simulink model "Controller"  (R2022b)
settings: Solver=FixedStepDiscrete  StartTime=0.0  StopTime=10.0  FixedStep=CONTROL_CONST.dt  MaxStep=CONTROL_PARAM.dt  RelTol=1e-3
values from neighbouring files (symbols this model uses):
  CONTROL_EXPORT = Simulink.Parameter(CONTROL_EXPORT_VALUE)    [control_model_init.m]
  CONTROL_PARAM = Simulink.Parameter(CONTROL_PARAM_VALUE)    [control_model_init.m]
undefined symbols (not defined in the file or in its folder): actuator_cmd, CONTROL_CONST, DiscIntNeverNeededParam, timestamp
libraries: simulink x3, FMT_Model_Lib x2, simulink_extras x2, drivingvehiclecontroller x2
settings Model: Creator=19114  LastModifiedBy=19114
settings OptimizationCC: DefaultParameterBehavior=Inlined  DefaultUnderspecifiedDataType=single  EnhancedBackFolding=on  PassReuseOutputArgsAs=Individual arguments  ZeroExternalMemoryAtStartup=off  ZeroInternalMemoryAtStartup=off  OptimizeBlockOrder=speed  DifferentSizesBufferReuse=on  OptimizationCustomize=off  EfficientTunableParamExpr=on
settings DebuggingCC: ParameterTunabilityLossMsg=error  UnconnectedInputMsg=warning  UnconnectedOutputMsg=warning  UnconnectedLineMsg=warning
settings HardwareCC: ProdBitPerPointer=32  ProdBitPerSizeT=32  ProdBitPerPtrDiffT=32  ProdLargestAtomicInteger=Long  ProdLargestAtomicFloat=Double  ProdWordSize=32  ProdHWDeviceType=ARM Compatible->ARM Cortex-M
settings ModelReferenceCC: EnableRefExpFcnMdlSchedulingChecks=on
settings SFSimCC: MATLABDynamicMemAlloc=off
settings RTWCC: Description=Embedded Coder  SystemTargetFile=ert.tlc  TemplateMakefile=ert_default_tmf  DLArmComputeVersion=19.05
settings CodeAppCC: ForceParamTrailComments=on  IgnoreCustomStorageClasses=off  OperatorAnnotations=on  SimulinkDataObjDesc=on  SFDataObjDesc=on  InsertBlockDesc=on
settings ERTTargetCC: TargetLangStandard=C99 (ISO)  GenerateSampleERTMain=on  SupportVariableSizeSignals=on  InlinedParameterPlacement=NonHierarchical  ERTCustomFileTemplate=example_file_process.tlc

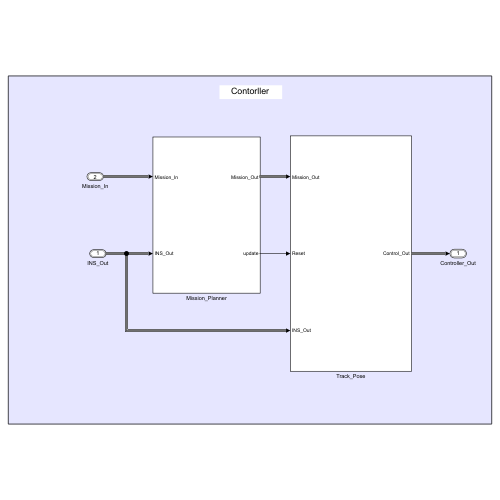
[thumbnail: Simulink's stored preview of the top-level diagram]
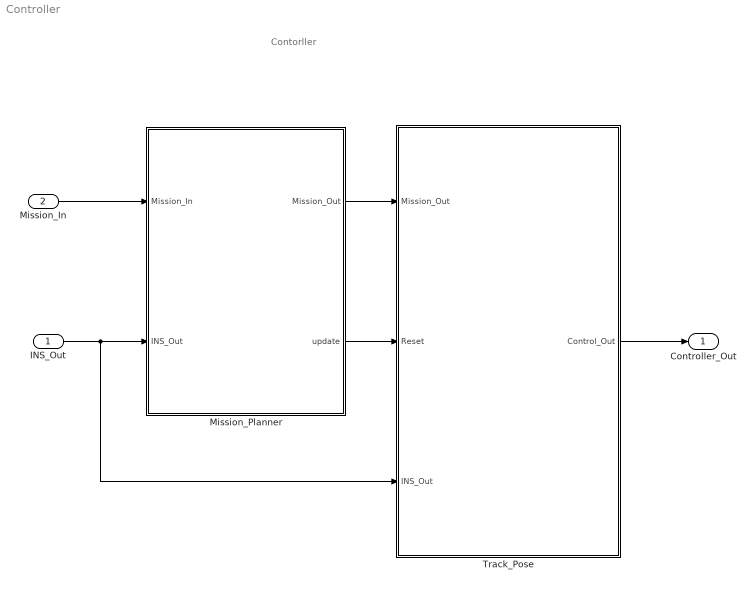
== system Controller ==
  note: Contorller
  INS_Out : Inport  OutDataTypeStr=Bus: INS_Out_Bus
  Mission_In : Inport  Port=2  OutDataTypeStr=Bus: Mission_Bus
  Mission_Planner : Subsystem
  Track_Pose : Subsystem
  Controller_Out : Outport  OutDataTypeStr=Bus: Control_Out_Bus
  wires:
  Track_Pose/1(Control_Out) -> Controller_Out/1
  Mission_Planner/1(Mission_Out) -> Track_Pose/1(Mission_Out)
  INS_Out/1 -> Mission_Planner/2(INS_Out), Track_Pose/3(INS_Out)
  Mission_In/1 -> Mission_Planner/1(Mission_In)
  Mission_Planner/2(update) -> Track_Pose/2(Reset)

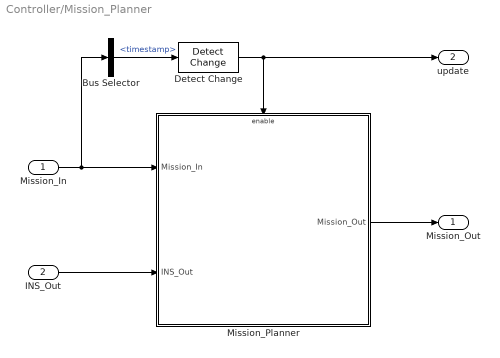
== system Controller/Mission_Planner ==
  Mission_In : Inport
  INS_Out : Inport  Port=2
  Bus Selector : BusSelector  OutputSignals=timestamp
  Detect Change : simulink/Logic and Bit Operations/Detect Change  vinit=0  OutDataTypeStr=boolean
  Mission_Planner : Subsystem
  Mission_Out : Outport
  update : Outport  Port=2
  wires:
  INS_Out/1 -> Mission_Planner/2(INS_Out)
  Mission_Planner/1(Mission_Out) -> Mission_Out/1
  Bus Selector/1 -> Detect Change/1  "<timestamp>"
  Mission_In/1 -> Bus Selector/1, Mission_Planner/1(Mission_In)
  Detect Change/1 -> Mission_Planner/Enable, update/1

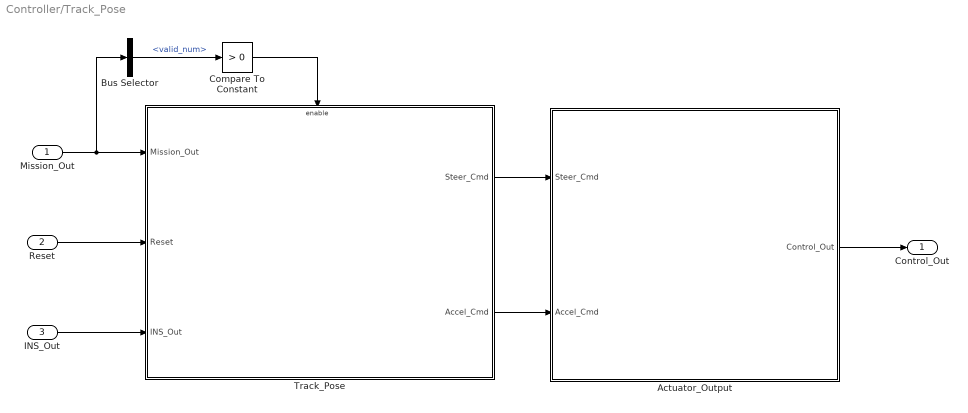
== system Controller/Track_Pose ==
  Mission_Out : Inport
  Reset : Inport  Port=2
  INS_Out : Inport  Port=3
  Actuator_Output : Subsystem
  Bus Selector : BusSelector  OutputSignals=valid_num
  Compare To Constant : simulink/Logic and Bit Operations/Compare To Constant  relop=>  const=0  OutDataTypeStr=boolean
  Track_Pose : Subsystem
  Control_Out : Outport
  wires:
  Reset/1 -> Track_Pose/2(Reset)
  Mission_Out/1 -> Bus Selector/1, Track_Pose/1(Mission_Out)
  INS_Out/1 -> Track_Pose/3(INS_Out)
  Bus Selector/1 -> Compare To Constant/1  "<valid_num>"
  Compare To Constant/1 -> Track_Pose/Enable
  Actuator_Output/1(Control_Out) -> Control_Out/1
  Track_Pose/1(Steer_Cmd) -> Actuator_Output/1(Steer_Cmd)
  Track_Pose/2(Accel_Cmd) -> Actuator_Output/2(Accel_Cmd)

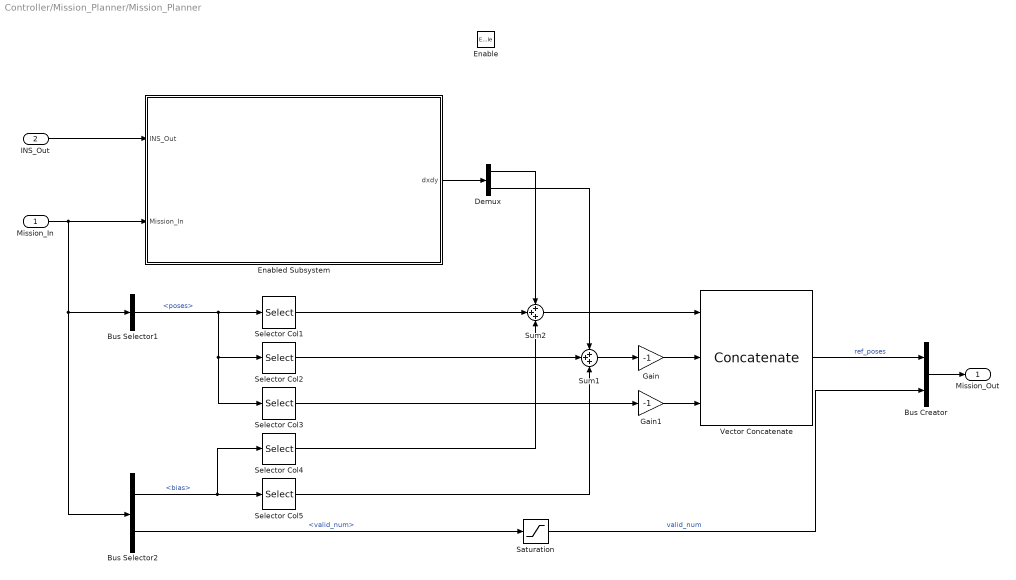
== system Controller/Mission_Planner/Mission_Planner ==
  Mission_In : Inport
  INS_Out : Inport  Port=2
  Enable : EnablePort
  Bus Creator : BusCreator  Inputs=2
  Bus Selector1 : BusSelector  OutputSignals=poses
  Bus Selector2 : BusSelector  OutputSignals=bias,valid_num
  Demux : Demux  Outputs=2
  Enabled Subsystem : Subsystem  TreatAsAtomicUnit=on
  Gain : Gain  Gain=-1
  Gain1 : Gain  Gain=-1
  Saturation : Saturate  UpperLimit=50  LowerLimit=0
  Selector Col1 : Selector  NumberOfDimensions=2  InputPortWidth=3  IndexOptions=Select all,Index vector (dialog)  Indices=[1 3],1  OutputSizes=1,1
  Selector Col2 : Selector  NumberOfDimensions=2  InputPortWidth=3  IndexOptions=Select all,Index vector (dialog)  Indices=[1 3],2  OutputSizes=1,1
  Selector Col3 : Selector  NumberOfDimensions=2  InputPortWidth=3  IndexOptions=Select all,Index vector (dialog)  Indices=[1 3],3  OutputSizes=1,1
  Selector Col4 : Selector  InputPortWidth=2  IndexOptions=Index vector (dialog)  Indices=[1]  OutputSizes=1
  Selector Col5 : Selector  InputPortWidth=2  IndexOptions=Index vector (dialog)  Indices=[1]  OutputSizes=1
  Sum1 : Sum  Inputs=+++
  Sum2 : Sum  Inputs=+++
  Vector Concatenate : Concatenate  NumInputs=3  Mode=Multidimensional array  ConcatenateDimension=2
  Mission_Out : Outport
  wires:
  Demux/1 -> Sum2/1
  Bus Selector1/1 -> Selector Col3/1, Selector Col2/1, Selector Col1/1  "<poses>"
  Demux/2 -> Sum1/1
  Selector Col3/1 -> Gain1/1
  Selector Col5/1 -> Sum1/3
  Bus Selector2/1 -> Selector Col4/1, Selector Col5/1  "<bias>"
  Mission_In/1 -> Bus Selector2/1, Bus Selector1/1, Enabled Subsystem/2(Mission_In)
  Saturation/1 -> Bus Creator/2  "valid_num"
  Vector Concatenate/1 -> Bus Creator/1  "ref_poses"
  Selector Col1/1 -> Sum2/2
  Enabled Subsystem/1(dxdy) -> Demux/1
  Selector Col2/1 -> Sum1/2
  Bus Selector2/2 -> Saturation/1  "<valid_num>"
  Selector Col4/1 -> Sum2/3
  Gain/1 -> Vector Concatenate/2
  Gain1/1 -> Vector Concatenate/3
  INS_Out/1 -> Enabled Subsystem/1(INS_Out)
  Sum1/1 -> Gain/1
  Sum2/1 -> Vector Concatenate/1
  Bus Creator/1 -> Mission_Out/1

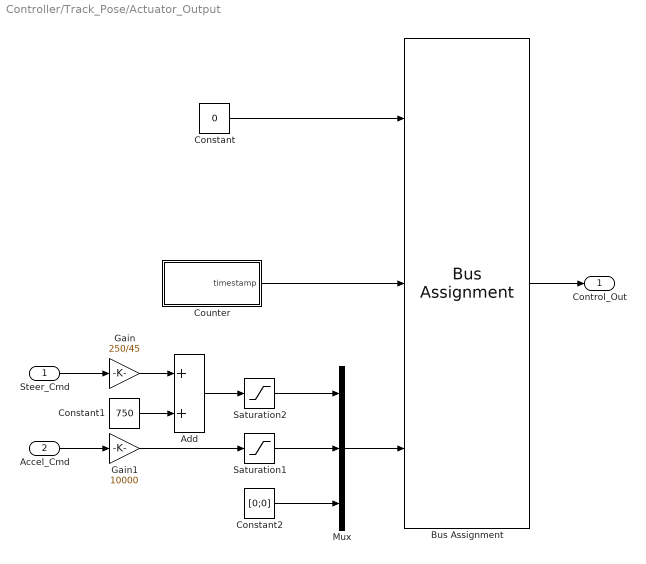
== system Controller/Track_Pose/Actuator_Output ==
  Steer_Cmd : Inport
  Accel_Cmd : Inport  Port=2
  Add : Sum
  Bus Assignment : BusAssignment  AssignedSignals=timestamp,actuator_cmd
  Constant : Constant  Value=0  OutDataTypeStr=Bus: Control_Out_Bus
  Constant1 : Constant  Value=750
  Constant2 : Constant  Value=[0;0]  OutDataTypeStr=int16
  Counter : Subsystem
  Gain : Gain  Gain=250/45
  Gain1 : Gain  Gain=10000
  Mux : Mux  Inputs=3
  Saturation1 : Saturate  UpperLimit=10000  LowerLimit=-10000  OutDataTypeStr=int16
  Saturation2 : Saturate  UpperLimit=1250  LowerLimit=250  OutDataTypeStr=int16
  Control_Out : Outport
  wires:
  Saturation2/1 -> Mux/1
  Steer_Cmd/1 -> Gain/1
  Saturation1/1 -> Mux/2
  Gain1/1 -> Saturation1/1
  Counter/1(timestamp) -> Bus Assignment/2
  Mux/1 -> Bus Assignment/3
  Constant2/1 -> Mux/3
  Constant1/1 -> Add/2
  Add/1 -> Saturation2/1
  Constant/1 -> Bus Assignment/1
  Gain/1 -> Add/1
  Bus Assignment/1 -> Control_Out/1
  Accel_Cmd/1 -> Gain1/1

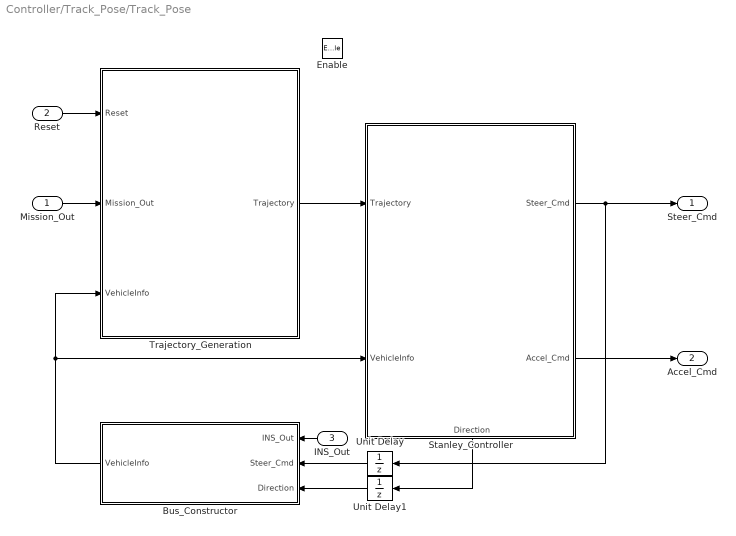
== system Controller/Track_Pose/Track_Pose ==
  Mission_Out : Inport
  Reset : Inport  Port=2
  INS_Out : Inport  Port=3
  Enable : EnablePort
  Bus_Constructor : Subsystem
  Stanley_Controller : Subsystem
      settings: PortSchema="{\"entries\":[{\"content\":{\"sides\":[{\"content\":{\"connectorIds\":[\"In1\",\"In2\"]},\"type\":\"ConnectorPlacement.EquallySpacedRectSide\",\"uuid\":\"cd03ad2f-d590-470d-91e9-617efa625f45\"},{\"content\":{\"connectorIds\":[\"Out1\",\"Out2\"],\"side\":\"RIGHT\"},\"type\":\"ConnectorPlacement.EquallySpacedRectSide\",\"uuid\":\"d63ae980-0075-4a72-87ac-5d939bfc1f03\"},{\"content\":{\"connectorIds\":[],\"side\":\"TOP\"},\"type\":\"ConnectorPlacement.EquallySpacedRectSide\",\"uuid\":\"29b7d5c8-9b77-4e8f-a72e-4b2a40d99676\"},{\"content\":{\"connectorIds\":[\"Out3\"],\"side\":\"BOTTOM\"},\"type\":\"ConnectorPlacement.EquallySpacedRectSide\",\"uuid\":\"d6191935-9086-4c4a-8544-60b3ebc96614\"}]},\"type\":\"ConnectorPlacement.EquallySpacedConnector\",\"uuid\":\"aed66183-a094-43c8-9c25-3324dbeb16c4\"}],\"packageUris\":[\"http://schema.mathworks.com/mf0/Connector/R2020b\"],\"version\":\"1.0\"}"
  Trajectory_Generation : Subsystem
  Unit Delay : UnitDelay  SampleTime=-1  HasFrameUpgradeWarning=on
  Unit Delay1 : UnitDelay  InitialCondition=1  SampleTime=-1  HasFrameUpgradeWarning=on
  Steer_Cmd : Outport
  Accel_Cmd : Outport  Port=2
  wires:
  Unit Delay1/1 -> Bus_Constructor/3(Direction)
  Mission_Out/1 -> Trajectory_Generation/2(Mission_Out)
  Stanley_Controller/3(Direction) -> Unit Delay1/1
  Unit Delay/1 -> Bus_Constructor/2(Steer_Cmd)
  Bus_Constructor/1(VehicleInfo) -> Trajectory_Generation/3(VehicleInfo), Stanley_Controller/2(VehicleInfo)
  INS_Out/1 -> Bus_Constructor/1(INS_Out)
  Trajectory_Generation/1(Trajectory) -> Stanley_Controller/1(Trajectory)
  Stanley_Controller/1(Steer_Cmd) -> Steer_Cmd/1, Unit Delay/1
  Reset/1 -> Trajectory_Generation/1(Reset)
  Stanley_Controller/2(Accel_Cmd) -> Accel_Cmd/1

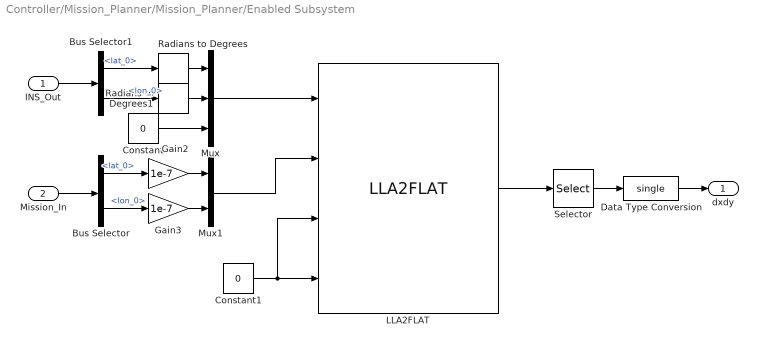
== system Controller/Mission_Planner/Mission_Planner/Enabled Subsystem ==
  INS_Out : Inport
  Mission_In : Inport  Port=2
  Bus Selector : BusSelector  OutputSignals=lat_0,lon_0
  Bus Selector1 : BusSelector  OutputSignals=lat_0,lon_0
  Constant : Constant  Value=0  OutDataTypeStr=double
  Constant1 : Constant  Value=0  OutDataTypeStr=double
  Data Type Conversion : DataTypeConversion  OutDataTypeStr=single  SaturateOnIntegerOverflow=off  RndMeth=Floor
  Gain2 : Gain  Gain=1e-7  OutDataTypeStr=double
  Gain3 : Gain  Gain=1e-7  OutDataTypeStr=double
  LLA2FLAT : FMT_Model_Lib/Transformation/LLA2FLAT
      settings: SourceProductName=FMT Toolbox
  Mux : Mux  Inputs=3
  Mux1 : Mux  Inputs=2
  Radians to Degrees : simulink_extras/Transformations/Radians to Degrees
  Radians to Degrees1 : simulink_extras/Transformations/Radians to Degrees
  Selector : Selector  InputPortWidth=3  IndexOptions=Index vector (dialog)  Indices=[1 2]  OutputSizes=1
  dxdy : Outport
  wires:
  Mux1/1 -> LLA2FLAT/2
  Constant/1 -> Mux/3
  Constant1/1 -> LLA2FLAT/3, LLA2FLAT/4
  Mission_In/1 -> Bus Selector/1
  INS_Out/1 -> Bus Selector1/1
  LLA2FLAT/1 -> Selector/1
  Bus Selector1/1 -> Radians to Degrees/1  "<lat_0>"
  Bus Selector1/2 -> Radians to Degrees1/1  "<lon_0>"
  Bus Selector/1 -> Gain2/1  "<lat_0>"
  Bus Selector/2 -> Gain3/1  "<lon_0>"
  Gain3/1 -> Mux1/2
  Gain2/1 -> Mux1/1
  Selector/1 -> Data Type Conversion/1
  Data Type Conversion/1 -> dxdy/1
  Mux/1 -> LLA2FLAT/1
  Radians to Degrees/1 -> Mux/1
  Radians to Degrees1/1 -> Mux/2

== system Controller/Track_Pose/Actuator_Output/Counter ==
  Data Type Conversion2 : DataTypeConversion  OutDataTypeStr=uint32  SaturateOnIntegerOverflow=off  RndMeth=Floor
  Memory1 : Memory
  Sum : Sum  Inputs=|++
  dt : Constant  Value=CONTROL_EXPORT.period  OutDataTypeStr=uint32
  timestamp : Outport
  wires:
  dt/1 -> Sum/1
  Sum/1 -> Memory1/1
  Data Type Conversion2/1 -> timestamp/1
  Memory1/1 -> Sum/2, Data Type Conversion2/1

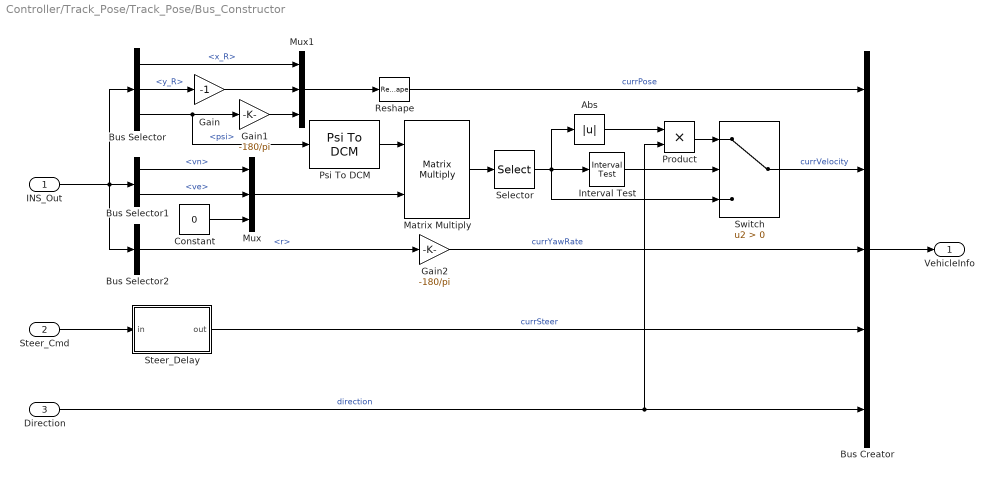
== system Controller/Track_Pose/Track_Pose/Bus_Constructor ==
  INS_Out : Inport
  Steer_Cmd : Inport  Port=2
  Direction : Inport  Port=3
  Abs : Abs  SaturateOnIntegerOverflow=off
  Bus Creator : BusCreator  Inputs=5  OutDataTypeStr=Bus: VehicheInfo_Bus
      settings: InheritFromInputs=off
  Bus Selector : BusSelector  OutputSignals=x_R,y_R,psi
  Bus Selector1 : BusSelector  OutputSignals=vn,ve
  Bus Selector2 : BusSelector  OutputSignals=r
  Constant : Constant  Value=0  OutDataTypeStr=single
  Gain : Gain  Gain=-1
  Gain1 : Gain  Gain=-180/pi
  Gain2 : Gain  Gain=-180/pi
  Interval Test : simulink/Logic and Bit Operations/Interval Test  IntervalClosedRight=on  uplimit=0.1  IntervalClosedLeft=on  lowlimit=-0.1  OutDataTypeStr=boolean
  Matrix Multiply : Product  Multiplication=Matrix(*)
  Mux : Mux  Inputs=3
  Mux1 : Mux  Inputs=3
  Product : Product
  Psi To DCM : FMT_Model_Lib/Transformation/Psi To DCM
      settings: SourceProductName=FMT Toolbox
  Reshape : Reshape  OutputDimensionality=Customize  OutputDimensions=[1,3]
  Selector : Selector  InputPortWidth=3  IndexOptions=Index vector (dialog)  Indices=[1]  OutputSizes=1
  Steer_Delay : Subsystem  mask{K=1, T=0.1}
      mask Display: disp('K/(1+Tz^{-1})', 'texmode', 'on')
  Switch : Switch  Criteria=u2 > Threshold  SaturateOnIntegerOverflow=off  InputSameDT=off
  VehicleInfo : Outport
  wires:
  Bus Creator/1 -> VehicleInfo/1
  Bus Selector1/1 -> Mux/1  "<vn>"
  Bus Selector1/2 -> Mux/2  "<ve>"
  Constant/1 -> Mux/3
  Bus Selector/3 -> Gain1/1, Psi To DCM/1  "<psi>"
  Psi To DCM/1 -> Matrix Multiply/1
  Mux/1 -> Matrix Multiply/2
  Matrix Multiply/1 -> Selector/1
  Mux1/1 -> Reshape/1
  Bus Selector/1 -> Mux1/1  "<x_R>"
  Bus Selector/2 -> Gain/1  "<y_R>"
  Gain/1 -> Mux1/2
  Gain1/1 -> Mux1/3
  INS_Out/1 -> Bus Selector/1, Bus Selector2/1, Bus Selector1/1
  Bus Selector2/1 -> Gain2/1  "<r>"
  Steer_Cmd/1 -> Steer_Delay/1(in)
  Steer_Delay/1(out) -> Bus Creator/4  "currSteer"
  Gain2/1 -> Bus Creator/3  "currYawRate"
  Reshape/1 -> Bus Creator/1  "currPose"
  Direction/1 -> Product/2, Bus Creator/5  "direction"
  Selector/1 -> Abs/1, Switch/3, Interval Test/1
  Interval Test/1 -> Switch/2
  Switch/1 -> Bus Creator/2  "currVelocity"
  Product/1 -> Switch/1
  Abs/1 -> Product/1

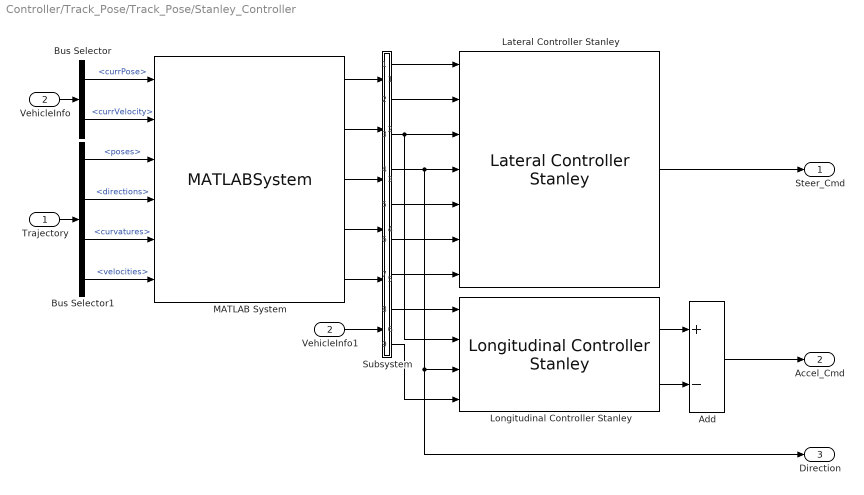
== system Controller/Track_Pose/Track_Pose/Stanley_Controller ==
  Trajectory : Inport
  VehicleInfo : Inport  Port=2
  Add : Sum  Inputs=+-
  Bus Selector : BusSelector  OutputSignals=currPose,currVelocity
  Bus Selector1 : BusSelector  OutputSignals=poses,directions,curvatures,velocities
  Lateral Controller Stanley : drivingvehiclecontroller/Lateral Controller Stanley  ModelType=Dynamic bicycle model  PositionGainF=2  PositionGainR=2.5  YawRateGain=0.25  DelayGain=0.2  VehicleMass=1  Lf=0.2  Lr=0.2  TireStiffness=19  Wheelbase=0.4  MaxSteeringAngle=30
  Longitudinal Controller Stanley : drivingvehiclecontroller/Longitudinal Controller Stanley  Kp=CONTROL_PARAM.KP  Ki=CONTROL_PARAM.KI  SampleTime=CONTROL_CONST.dt  MaxAcceleration=20  MaxDeceleration=20
  MATLAB System : MATLABSystem  System=HelperPathAnalyzer  Wheelbase=0.4  HasResetOutput=on  SimulateUsing=Code generation
      mask Type: HelperPathAnalyzer
      mask Display:
      | disp(['Helper' char(10) 'Path' char(10) 'Analyzer']);
      | port_label('input',1,'CurrPose');
      | port_label('input',2,'CurrVelocity');
      | port_label('input',3,'RefPoses');
      | port_label('input',4,'Directions');
      | port_label('input',5,'Curvatures');
      | port_label('input',6,'RefVelocities');
      | port_label('output',1,'RefPose');
      | port_label('output',2,'RefVelocity');
      | port_label('output',3,'Direction');
      | port_label('output',4,'Curvature');
      | port_label('output',5,'Reset');
  Subsystem : Subsystem
  VehicleInfo1 : InportShadow  Port=2
  Steer_Cmd : Outport
  Accel_Cmd : Outport  Port=2
  Direction : Outport  Port=3
  wires:
  MATLAB System/5 -> Subsystem/5(Reset)
  Subsystem/9(Reset1) -> Longitudinal Controller Stanley/4
  Bus Selector1/3 -> MATLAB System/5  "<curvatures>"
  Subsystem/3(CurrVelocity) -> Longitudinal Controller Stanley/2, Lateral Controller Stanley/3
  MATLAB System/4 -> Subsystem/4(Curvature)
  Subsystem/4(Direction1) -> Direction/1, Longitudinal Controller Stanley/3, Lateral Controller Stanley/4
  Bus Selector1/4 -> MATLAB System/6  "<velocities>"
  VehicleInfo1/1 -> Subsystem/6(VehicleInfo)
  Trajectory/1 -> Bus Selector1/1
  VehicleInfo/1 -> Bus Selector/1
  Longitudinal Controller Stanley/2 -> Add/2
  Bus Selector1/2 -> MATLAB System/4  "<directions>"
  Subsystem/1(RefPose1) -> Lateral Controller Stanley/1
  Subsystem/8(RefVelocity1) -> Longitudinal Controller Stanley/1
  Subsystem/2(CurrPose) -> Lateral Controller Stanley/2
  Bus Selector/2 -> MATLAB System/2  "<currVelocity>"
  MATLAB System/1 -> Subsystem/1(RefPose)
  Longitudinal Controller Stanley/1 -> Add/1
  MATLAB System/3 -> Subsystem/3(Direction)
  MATLAB System/2 -> Subsystem/2(RefVelocity)
  Bus Selector1/1 -> MATLAB System/3  "<poses>"
  Bus Selector/1 -> MATLAB System/1  "<currPose>"
  Subsystem/5(Curvature1) -> Lateral Controller Stanley/5
  Subsystem/6(CurrYawRate) -> Lateral Controller Stanley/6
  Subsystem/7(CurrSteer) -> Lateral Controller Stanley/7
  Lateral Controller Stanley/1 -> Steer_Cmd/1
  Add/1 -> Accel_Cmd/1

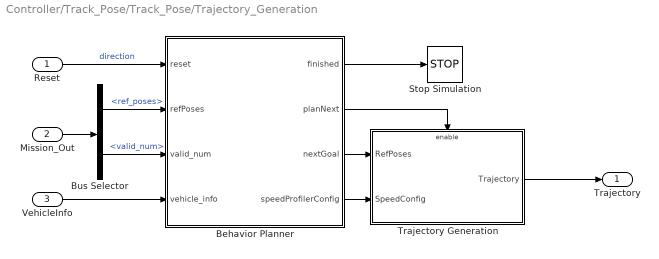
== system Controller/Track_Pose/Track_Pose/Trajectory_Generation ==
  Reset : Inport
  Mission_Out : Inport  Port=2
  VehicleInfo : Inport  Port=3
  Behavior Planner : MATLAB Function  TreatAsAtomicUnit=on
  Bus Selector : BusSelector  OutputSignals=ref_poses,valid_num
  Stop Simulation : Stop
  Trajectory Generation : Subsystem
  Trajectory : Outport
  wires:
  Mission_Out/1 -> Bus Selector/1
  Behavior Planner/3(nextGoal) -> Trajectory Generation/1(RefPoses)
  Behavior Planner/4(speedProfilerConfig) -> Trajectory Generation/2(SpeedConfig)
  Bus Selector/1 -> Behavior Planner/2(refPoses)  "<ref_poses>"
  Bus Selector/2 -> Behavior Planner/3(valid_num)  "<valid_num>"
  VehicleInfo/1 -> Behavior Planner/4(vehicle_info)
  Trajectory Generation/1(Trajectory) -> Trajectory/1
  Behavior Planner/2(planNext) -> Trajectory Generation/Enable
  Reset/1 -> Behavior Planner/1(reset)  "direction"
  Behavior Planner/1(finished) -> Stop Simulation/1

== system Controller/Track_Pose/Track_Pose/Bus_Constructor/Steer_Delay ==
  in : Inport
  Discrete-Time Integrator : DiscreteIntegrator  gainval=K  SampleTime=-1  ICPrevOutput=DiscIntNeverNeededParam  ICPrevScaledInput=DiscIntNeverNeededParam
  Gain : Gain  Gain=1/T
  Subtract : Sum  Inputs=+-
  out : Outport  VectorParamsAs1DForOutWhenUnconnected=off
  wires:
  in/1 -> Subtract/1
  Subtract/1 -> Gain/1
  Gain/1 -> Discrete-Time Integrator/1
  Discrete-Time Integrator/1 -> Subtract/2, out/1

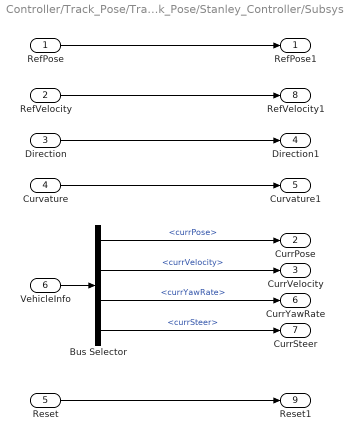
== system Controller/Track_Pose/Track_Pose/Stanley_Controller/Subsystem ==
  RefPose : Inport
  RefVelocity : Inport  Port=2
  Direction : Inport  Port=3
  Curvature : Inport  Port=4
  Reset : Inport  Port=5
  VehicleInfo : Inport  Port=6
  Bus Selector : BusSelector  OutputSignals=currPose,currVelocity,currYawRate,currSteer
  RefPose1 : Outport
  CurrPose : Outport  Port=2
  CurrVelocity : Outport  Port=3
  Direction1 : Outport  Port=4
  Curvature1 : Outport  Port=5
  CurrYawRate : Outport  Port=6
  CurrSteer : Outport  Port=7
  RefVelocity1 : Outport  Port=8
  Reset1 : Outport  Port=9
  wires:
  RefPose/1 -> RefPose1/1
  VehicleInfo/1 -> Bus Selector/1
  Bus Selector/1 -> CurrPose/1  "<currPose>"
  Bus Selector/2 -> CurrVelocity/1  "<currVelocity>"
  RefVelocity/1 -> RefVelocity1/1
  Curvature/1 -> Curvature1/1
  Bus Selector/3 -> CurrYawRate/1  "<currYawRate>"
  Bus Selector/4 -> CurrSteer/1  "<currSteer>"
  Reset/1 -> Reset1/1
  Direction/1 -> Direction1/1

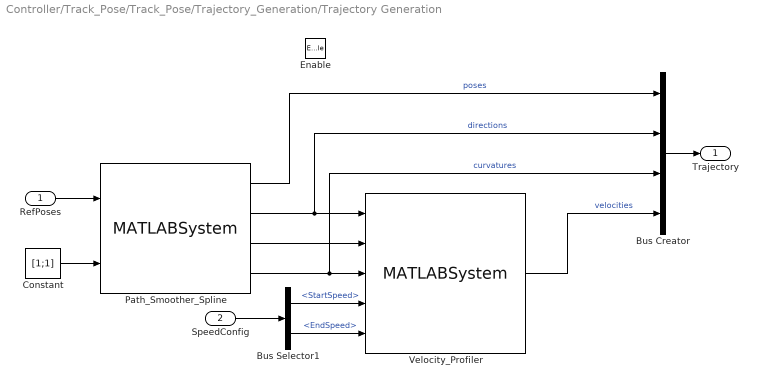
== system Controller/Track_Pose/Track_Pose/Trajectory_Generation/Trajectory Generation ==
  RefPoses : Inport
  SpeedConfig : Inport  Port=2
  Enable : EnablePort
  Bus Creator : BusCreator  Inputs=4
  Bus Selector1 : BusSelector  OutputSignals=StartSpeed,EndSpeed
  Constant : Constant  Value=[1;1]  OutDataTypeStr=Inherit: Inherit via back propagation
  Path_Smoother_Spline : MATLABSystem  System=PathSmootherSpline  NumSmoothPoses=CONTROL_CONST.NumOfPoints  MinSeparation=1e-3  SampleTime=-1  ShowOptionalOutports=on  SimulateUsing=Code generation
      mask Type: PathSmootherSpline
      mask Display:
      | disp(['Path' char(10) 'Smoother' char(10) 'Spline']);
      | port_label('input',1,'RefPoses');
      | port_label('input',2,'RefDirections');
      | port_label('output',1,'Poses');
      | port_label('output',2,'Directions');
      | port_label('output',3,'CumLengths');
      | port_label('output',4,'Curvatures');
  Velocity_Profiler : MATLABSystem  System=VelocityProfiler  MaxLongitudinalAccel=20  MaxLongitudinalDecel=20  MaxSpeed=20  MaxLongitudinalJerk=10  MaxLateralAccel=20  ShowOptionalOutport=off  SampleTime=-1  SimulateUsing=Code generation
      mask Type: VelocityProfiler
      mask Display:
      | disp(['Velocity' char(10) 'Profiler']);
      | port_label('input',1,'Directions');
      | port_label('input',2,'CumLengths');
      | port_label('input',3,'Curvatures');
      | port_label('input',4,'StartVelocity');
      | port_label('input',5,'EndVelocity');
      | port_label('output',1,'Velocities');
  Trajectory : Outport
  wires:
  Path_Smoother_Spline/2 -> Bus Creator/2, Velocity_Profiler/1  "directions"
  Path_Smoother_Spline/4 -> Bus Creator/3, Velocity_Profiler/3  "curvatures"
  Bus Selector1/2 -> Velocity_Profiler/5  "<EndSpeed>"
  RefPoses/1 -> Path_Smoother_Spline/1
  Bus Selector1/1 -> Velocity_Profiler/4  "<StartSpeed>"
  Path_Smoother_Spline/3 -> Velocity_Profiler/2
  Constant/1 -> Path_Smoother_Spline/2
  SpeedConfig/1 -> Bus Selector1/1
  Bus Creator/1 -> Trajectory/1
  Velocity_Profiler/1 -> Bus Creator/4  "velocities"
  Path_Smoother_Spline/1 -> Bus Creator/1  "poses"

== matlab function Controller/Track_Pose/Track_Pose/Trajectory_Generation/Behavior Planner ==
  data: finished output; reset input; planNext output; refPoses input; valid_num input; vehicle_info input Bus: VehicheInfo_Bus; nextGoal output; speedProfilerConfig output Bus: SpeedConfig_Bus
function [finished,planNext, nextGoal, speedProfilerConfig] = ...
    behaviorPlanning(reset, refPoses, valid_num, vehicle_info)

%behaviorPlanning generate navigation tasks and configurations for the 
%   Motion Planner block and the Trajectory Generator block.
nextGoal   = coder.nullcopy(zeros(2, 3, 'single')); %#ok<*NASGU>
planNext   = false; 

persistent goalIndex finalReached endSpeed
persistent nextGoalPose speedConfig

if isempty(goalIndex) || reset > 0
    % Initialize pose and speed
    finalReached = false;
    endSpeed  = single(1);
    goalIndex = 1;
    nextGoalPose = [vehicle_info.currPose ;refPoses(goalIndex,:)];
    speedConfig.StartSpeed  = vehicle_info.currVelocity;
    speedConfig.EndSpeed    = endSpeed;
    goalIndex = goalIndex + 1;
    planNext = true;
end


if ~finalReached
    % Plan a new path when reaching the goal
    if helperGoalChecker(nextGoalPose(end, :), vehicle_info.currPose, vehicle_info.currVelocity, speedConfig.EndSpeed, vehicle_info.direction)
        if goalIndex <= valid_num
            nextGoalPose = [refPoses(goalIndex,:) ;refPoses(goalIndex+1,:)];
            speedConfig.StartSpeed  = vehicle_info.currVelocity;
            speedConfig.EndSpeed    = endSpeed;
            goalIndex = goalIndex + 1;
            planNext = true;
        else
            % reach the last goal, clear setting pose and velocity.
            nextGoalPose(:, :) = single(0);
            speedConfig.StartSpeed = single(0);
            speedConfig.EndSpeed = single(0);
            finalReached       = true;
        end
    end
end
    
nextGoal            = nextGoalPose;
speedProfilerConfig = speedConfig;
finished            = finalReached;
end
